simulink model "model1"  (R2024a)
settings: Solver=ode23t  StartTime=0.0  StopTime=finalatt{end,1}  MaxStep=0.1  RelTol=1e-3
undefined symbols (not defined in the file): finalatt, FrontAxle, FrontGear, MassWheel, NewData, RadiusWheel, RearAxle, RearGear, SlipAngle, TrackData, VehicleMass
libraries: fl_lib x16, batt_lib x13, nesl_utility x11, sdl_lib x7, ee_lib x2, simulink x1
(part 1 of 2)
settings Model: Creator=baiqu  LastModifiedBy=baiqu
settings SolverCC: MaxConsecutiveMinStep=5  ZeroCrossAlgorithm=Adaptive

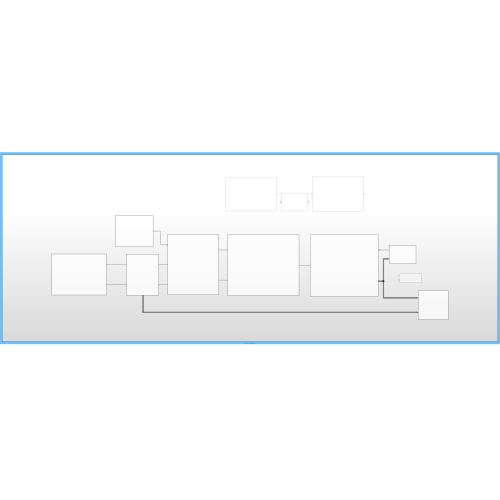
[thumbnail: Simulink's stored preview of the top-level diagram]
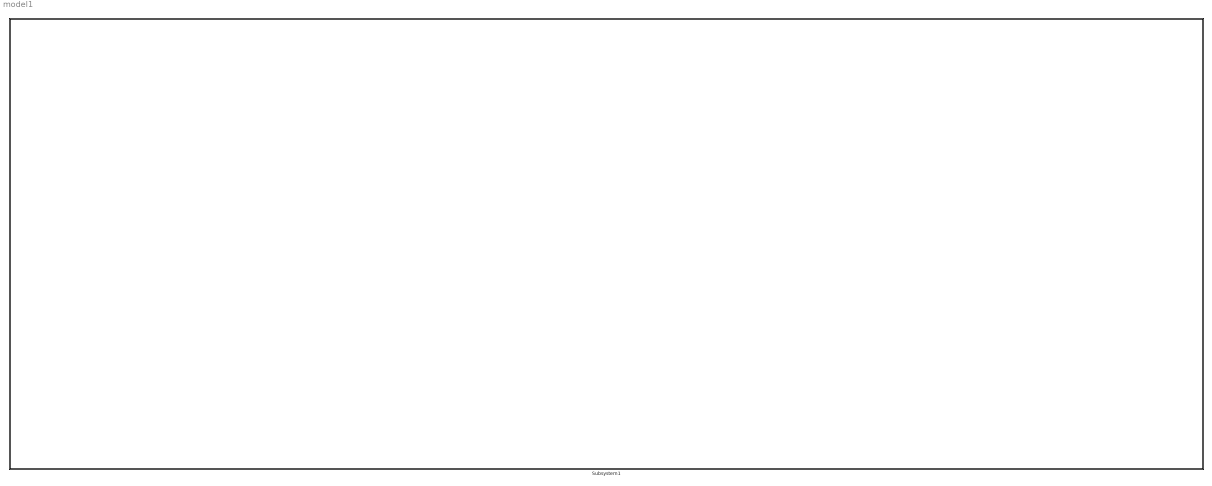
== system model1 ==
  Subsystem1 : Subsystem

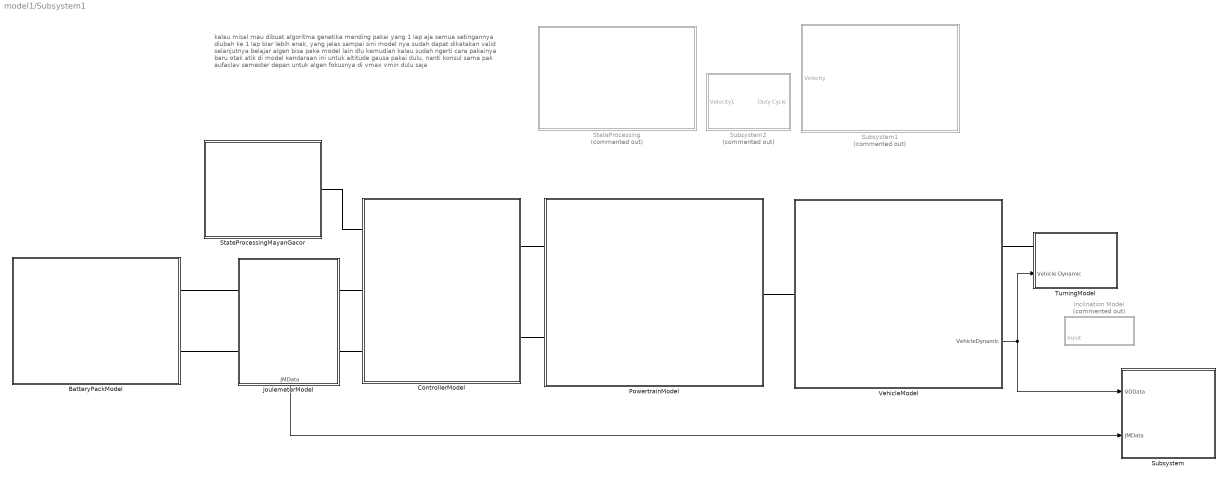
== system model1/Subsystem1 ==
  note: kalau misal mau dibuat algoritma genetika mending pakai yang 1 lap aja semua setingannya diubah ke 1 lap biar lebih enak, yang jelas sampai sini model nya sudah dapat dikatakan valid
      |
      | selanjutnya belajar algen bisa pake model lain dlu kemudian kalau sudah ngerti cara pakainya baru otak atik di model kendaraan ini
      |
      | untuk altitude gausa pakai dulu, nanti konsul sama pak aufaclav semester depan
      |
      | untuk algen fokusnya di vmax vmin dulu saja
  BatteryPackModel : Subsystem
  ControllerModel : Subsystem
  Inclination Model : Subsystem  Commented=on
      settings: PortSchema="{\"entries\":[{\"content\":{\"sides\":[{\"content\":{},\"type\":\"ConnectorPlacement.EquallySpacedRectSide\",\"uuid\":\"136e15b9-992d-4bd3-9ecd-22bc584851ec\"},{\"content\":{\"connectorIds\":[\"RConn1\",\"In1\"],\"side\":\"RIGHT\"},\"type\":\"ConnectorPlacement.EquallySpacedRectSide\",\"uuid\":\"21901198-73a1-4f2b-bd2a-55a4ec918fc9\"},{\"content\":{\"side\":\"TOP\"},\"type\":\"ConnectorPlacement.EquallySpacedRectSide\",\"uuid\":\"96b62914-b1ee-40c2-9187-7fe30b0e8d87\"}]},\"type\":\"ConnectorPlacement.EquallySpacedConnector\",\"uuid\":\"3de7d7f5-6cf3-49e2-811a-f65baadaba13\"}],\"packageUris\":[\"http://schema.mathworks.com/mf0/Connector/R2020b\"],\"version\":\"1.0\"}"
  JoulemeterModel : Subsystem
      settings: PortSchema="{\"entries\":[{\"content\":{\"sides\":[{\"content\":{\"connectorIds\":[\"LConn1\",\"LConn2\"]},\"type\":\"ConnectorPlacement.EquallySpacedRectSide\",\"uuid\":\"5b7f183a-bf7a-4999-b582-2617b2cbf3b5\"},{\"content\":{\"connectorIds\":[\"RConn1\",\"RConn2\"],\"side\":\"RIGHT\"},\"type\":\"ConnectorPlacement.EquallySpacedRectSide\",\"uuid\":\"60e6a297-a548-4f80-bd0a-fa1cc363ffaf\"},{\"content\":{\"side\":\"TOP\"},\"type\":\"ConnectorPlacement.EquallySpacedRectSide\",\"uuid\":\"7f0257a8-d3f8-4392-a80f-b293aa05a497\"},{\"content\":{\"connectorIds\":[\"Out1\"],\"side\":\"BOTTOM\"},\"type\":\"ConnectorPlacement.EquallySpacedRectSide\",\"uuid\":\"bc8eaeec-fb49-4b5e-9f30-46577002e429\"}]},\"type\":\"ConnectorPlacement.EquallySpacedConnector\",\"uuid\":\"4d471f89-f217-48cc-a8db-ea855d9b8dd6\"}],\"packageUris\":[\"http://schema.mathworks.com/mf0/Connector/R2020b\"],\"version\":\"1.0\"}"
  PowertrainModel : Subsystem
  StateProcessing : Subsystem  Commented=on
  StateProcessingMayanGacor : Subsystem
  Subsystem : Subsystem
  Subsystem1 : Subsystem  Commented=on
  Subsystem2 : Subsystem  Commented=on
  TurningModel : Subsystem
      settings: PortSchema="{\"entries\":[{\"content\":{\"sides\":[{\"content\":{\"connectorIds\":[\"LConn1\",\"In1\"]},\"type\":\"ConnectorPlacement.EquallySpacedRectSide\",\"uuid\":\"71e7bed3-e1e3-4832-b1c1-24de9e1463fb\"},{\"content\":{\"side\":\"RIGHT\"},\"type\":\"ConnectorPlacement.EquallySpacedRectSide\",\"uuid\":\"85b25ef4-cea1-4d54-8b2c-2c7e7889f274\"},{\"content\":{\"side\":\"TOP\"},\"type\":\"ConnectorPlacement.EquallySpacedRectSide\",\"uuid\":\"88c22c9a-8431-4448-acf4-309695bed040\"}]},\"type\":\"ConnectorPlacement.EquallySpacedConnector\",\"uuid\":\"9b68c14c-70b8-4970-8604-5181bbf23f66\"}],\"packageUris\":[\"http://schema.mathworks.com/mf0/Connector/R2020b\"],\"version\":\"1.0\"}"
  VehicleModel : Subsystem
      settings: PortSchema="{\"entries\":[{\"content\":{\"sides\":[{\"content\":{\"connectorIds\":[\"LConn1\"]},\"type\":\"ConnectorPlacement.EquallySpacedRectSide\",\"uuid\":\"dbac9918-d97a-4fb9-bcac-715c55eb3548\"},{\"content\":{\"connectorIds\":[\"RConn1\",\"Out1\"],\"side\":\"RIGHT\"},\"type\":\"ConnectorPlacement.EquallySpacedRectSide\",\"uuid\":\"c709c379-adcf-4afd-bad7-556514c49845\"},{\"content\":{\"side\":\"TOP\"},\"type\":\"ConnectorPlacement.EquallySpacedRectSide\",\"uuid\":\"0d093c29-8fc7-4ed3-9b38-7f716bf50260\"}]},\"type\":\"ConnectorPlacement.EquallySpacedConnector\",\"uuid\":\"a77c3579-3db4-497e-9cef-798accda3f16\"}],\"packageUris\":[\"http://schema.mathworks.com/mf0/Connector/R2020b\"],\"version\":\"1.0\"}"
  wires:
  JoulemeterModel/1(JMData) -> Subsystem/2(JMData)
  VehicleModel/1(VehicleDynamic) -> TurningModel/1(Vehicle Dynamic), Subsystem/1(VDData)
  connections:
  PowertrainModel/RConn1 -- VehicleModel/LConn1
  JoulemeterModel/LConn1 -- BatteryPackModel/RConn1
  ControllerModel/RConn1 -- PowertrainModel/LConn1
  JoulemeterModel/RConn2 -- ControllerModel/LConn3
  JoulemeterModel/RConn1 -- ControllerModel/LConn2
  PowertrainModel/LConn2 -- ControllerModel/RConn2
  BatteryPackModel/RConn2 -- JoulemeterModel/LConn2
  TurningModel/LConn1 -- VehicleModel/RConn1
  StateProcessingMayanGacor/RConn1 -- ControllerModel/LConn1

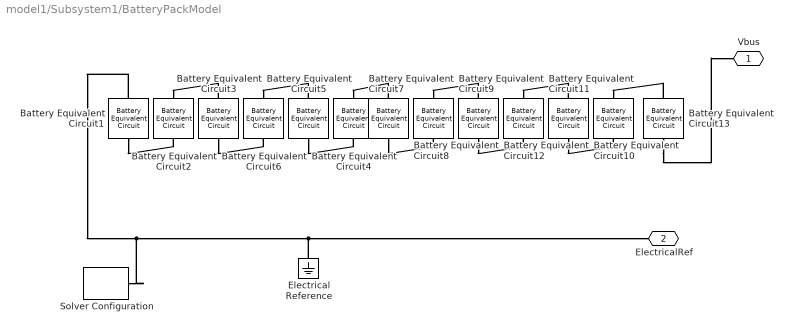
== system model1/Subsystem1/BatteryPackModel ==
  Battery Equivalent Circuit{1..13} (13 alike) : batt_lib/Cells/Battery Equivalent Circuit  Tag={'toolbox/physmod/battery/library/m/batt_lib_parts';'Cells/Battery_Equivalent_Circuit/Molicel/INR_21700_P45B.xml'}  BatteryCapacity=4.493 hr*A  ThermalModel=simscape.battery.enum.cells.BatteryThermalModel.ConstantTemperature  ExtrapolationMethod=simscape.enum.extrapolation.linear  EnableFaultExotherm=false % Parameter not set  TriggerTemperature=350 % Parameter not set K  SOCBreakpoints=[0 0.01 0.02 0.03 0.04 0.05 0.06 0.07 0.08 0.09 0.1 0.11 0.12 0.13 0.14 0.15 0.16 0.17 0.18 0.19 0.2 0.21 0.22 0.23 0.24 0.25 0.26 0.27 0.28 0.29 0.3 0.31 0.32 0.33 0.34 0.35 0.36 0.37 0.38 0.39 0.4 0.41 0.42 0.43 0.44 0.45 0.46 0.47 0.48 0.49 0.5 0.51 0.52 0.53 0.54 0.55 0.56 0.57 0.58 0.59 0.6 0.61 0.62 0.63 0.64 0.65 0.66 0.67 0.68 0.69 0.7 0.71 0.72 0.73 0.74 0.75 0.76 0.77 0.78 0.79 0.8 0.81 0.82 0.83 0.84 0.85 0.86 0.87 0.88 0.89 0.9 0.91 0.92 0.93 0.94 0.95 0.96 0.97 0.98 0.99 1]  TemperatureBreakpoints=[-40 -30 -20 0 23 45 60] degC  OpenCircuitVoltage=[3.17242 3.18272 3.19302 3.20331 3.21361 3.22391 3.23421 3.24451 3.25481 3.2651 3.2754 3.2857 3.296 3.3063 3.31659 3.32689 3.33719 3.34749 3.35779 3.36809 3.37838 3.38868 3.39898 3.40928 3.41958 3.42988 3.44017 3.45047 3.46077 3.47107 3.48137 3.49166 3.50196 3.51226 3.52256 3.53286 3.54316 3.55345 3.56375 3.57405 3.58435 3.59465 3.60495 3.61524 3.62554 3.63584 3.64614 3.65644 3.66673 3.67703 3.68733 3.69763 3.71041 3.72113 3.72997 3.73882 3.74912 3.75936 3.76951 3.7791 3.78865 3.79787 3.80709 3.8161 3.82509 3.83409 3.84308 3.85207 3.86107 3.87006 3.87901 3.88831 3.89824 3.90887 3.91951 3.93012 3.94073 3.95138 3.96184 3.97226 3.98268 3.99311 4.0032 4.01221 4.01944 4.02668 4.03286 4.03874 4.04383 4.0488 4.05377 4.05873 4.06312 4.06753 4.07333 4.08117 4.08904 4.09911 4.11111 4.13802 4.16831] V  OpenCircuitVoltageThermal=[3.17242 3.17242 3.17242 3.17242 3.17242 3.17242 3.17242;3.18272 3.18272 3.18272 3.18272 3.18272 3.18272 3.18272;3.19302 3.19302 3.19302 3.19302 3.19302 3.19302 3.19302;3.20331 3.20331 3.20331 3.20331 3.20331 3.20331 3.20331;3.21361 3.21361 3.21361 3.21361 3.21361 3.21361 3.21361;3.22391 3.22391 3.22391 3.22391 3.22391 3.22391 3.22391;3.23421 3.23421 3.23421 3.23421 3.23421 3.23421 3.23421;3.24451 3.24451 3.24451 3.24451 3.24451 3.24451 3.24451;3.25481 3.25481 3.25481 3.25481 3.25481 3.25481 3.25481;3.2651 3.2651 3.2651 3.2651 3.2651 3.2651 3.2651;3.2754 3.2754 3.2754 3.2754 3.2754 3.2754 3.2754;3.2857 3.2857 3.2857 3.2857 3.2857 3.2857 3.2857;3.296 3.296 3.296 3.296 3.296 3.296 3.296;3.3063 3.3063 3.3063 3.3063 3.3063 3.3063 3.3063;3.31659 3.31659 3.31659 3.31659 3.31659 3.31659 3.31659;3.32689 3.32689 3.32689 3.32689 3.32689 3.32689 3.32689;3.33719 3.33719 3.33719 3.33719 3.33719 3.33719 3.33719;3.34749 3.34749 3.34749 3.34749 3.34749 3.34749 3.34749;3.35779 3.35779 3.35779 3.35779 3.35779 3.35779 3.35779;3.36809 3.36809 3.36809 3.36809 3.36809 3.36809 3.36809;3.37838 3.37838 3.37838 3.37838 3.37838 3.37838 3.37838;3.38868 3.38868 3.38868 3.38868 3.38868 3.38868 3.38868;3.39898 3.39898 3.39898 3.39898 3.39898 3.39898 3.39898;3.40928 3.40928 3.40928 3.40928 3.40928 3.40928 3.40928;3.41958 3.41958 3.41958 3.41958 3.41958 3.41958 3.41958;3.42988 3.42988 3.42988 3.42988 3.42988 3.42988 3.42988;3.44017 3.44017 3.44017 3.44017 3.44017 3.44017 3.44017;3.45047 3.45047 3.45047 3.45047 3.45047 3.45047 3.45047;3.46077 3.46077 3.46077 3.46077 3.46077 3.46077 3.46077;3.47107 3.47107 3.47107 3.47107 3.47107 3.47107 3.47107;3.48137 3.48137 3.48137 3.48137 3.48137 3.48137 3.48137;3.49166 3.49166 3.49166 3.49166 3.49166 3.49166 3.49166;3.50196 3.50196 3.50196 3.50196 3.50196 3.50196 3.50196;3.51226 3.51226 3.51226 3.51226 3.51226 3.51226 3.51226;3.52256 3.52256 3.52256 3.52256 3.52256 3.52256 3.52256;3.53286 3.53286 3.53286 3.53286 3.53286 3.53286 3.53286;3.54316 3.54316 3.54316 3.54316 3.54316 3.54316 3.54316;3.55345 3.55345 3.55345 3.55345 3.55345 3.55345 3.55345;3.56375 3.56375 3.56375 3.56375 3.56375 3.56375 3.56375;3.57405 3.57405 3.57405 3.57405 3.57405 3.57405 3.57405;3.58435 3.58435 3.58435 3.58435 3.58435 3.58435 3.58435;3.59465 3.59465 3.59465 3.59465 3.59465 3.59465 3.59465;3.60495 3.60495 3.60495 3.60495 3.60495 3.60495 3.60495;3.61524 3.61524 3.61524 3.61524 3.61524 3.61524 3.61524;3.62554 3.62554 3.62554 3.62554 3.62554 3.62554 3.62554;3.63584 3.63584 3.63584 3.63584 3.63584 3.63584 3.63584;3.64614 3.64614 3.64614 3.64614 3.64614 3.64614 3.64614;3.65644 3.65644 3.65644 3.65644 3.65644 3.65644 3.65644;3.66673 3.66673 3.66673 3.66673 3.66673 3.66673 3.66673;3.67703 3.67703 3.67703 3.67703 3.67703 3.67703 3.67703;3.68733 3.68733 3.68733 3.68733 3.68733 3.68733 3.68733;3.69763 3.69763 3.69763 3.69763 3.69763 3.69763 3.69763;3.71041 3.71041 3.71041 3.71041 3.71041 3.71041 3.71041;3.72113 3.72113 3.72113 3.72113 3.72113 3.72113 3.72113;3.72997 3.72997 3.72997 3.72997 3.72997 3.72997 3.72997;3.73882 3.73882 3.73882 3.73882 3.73882 3.73882 3.73882;3.74912 3.74912 3.74912 3.74912 3.74912 3.74912 3.74912;3.75936 3.75936 3.75936 3.75936 3.75936 3.75936 3.75936;3.76951 3.76951 3.76951 3.76951 3.76951 3.76951 3.76951;3.7791 3.7791 3.7791 3.7791 3.7791 3.7791 3.7791;3.78865 3.78865 3.78865 3.78865 3.78865 3.78865 3.78865;3.79787 3.79787 3.79787 3.79787 3.79787 3.79787 3.79787;3.80709 3.80709 3.80709 3.80709 3.80709 3.80709 3.80709;3.8161 3.8161 3.8161 3.8161 3.8161 3.8161 3.8161;3.82509 3.82509 3.82509 3.82509 3.82509 3.82509 3.82509;3.83409 3.83409 3.83409 3.83409 3.83409 3.83409 3.83409;3.84308 3.84308 3.84308 3.84308 3.84308 3.84308 3.84308;3.85207 3.85207 3.85207 3.85207 3.85207 3.85207 3.85207;3.86107 3.86107 3.86107 3.86107 3.86107 3.86107 3.86107;3.87006 3.87006 3.87006 3.87006 3.87006 3.87006 3.87006;3.87901 3.87901 3.87901 3.87901 3.87901 3.87901 3.87901;3.88831 3.88831 3.88831 3.88831 3.88831 3.88831 3.88831;3.89824 3.89824 ...(+1594 chars)] V  VoltageRange=[2.25 Inf] V  HysteresisModel=simscape.battery.enum.cells.HysteresisModel.none  MaximumHysteresisVoltage=[0, 0, 0, 0, 0, 0, 0] % Parameter not set V  InstantaneousHysteresisVoltage=[0, 0, 0, 0, 0, 0, 0] % Parameter not set V  HysteresisRate=0.1 % Parameter not set  MaximumHysteresisVoltageThermal=[0, 0, 0; 0, 0, 0; 0, 0, 0; 0, 0, 0; 0, 0, 0; 0, 0, 0; 0, 0, 0] % Parameter not set V  InstantaneousHysteresisVoltageThermal=[0, 0, 0; 0, 0, 0; 0, 0, 0; 0, 0, 0; 0, 0, 0; 0, 0, 0; 0, 0, 0] % Parameter not set V  HysteresisRateThermal=0.1 % Parameter not set  ResistanceSOCBreakpoints=[0 0.01 0.02 0.03 0.04 0.05 0.06 0.07 0.08 0.09 0.1 0.11 0.12 0.13 0.14 0.15 0.16 0.17 0.18 0.19 0.2 0.21 0.22 0.23 0.24 0.25 0.26 0.27 0.28 0.29 0.3 0.31 0.32 0.33 0.34 0.35 0.36 0.37 0.38 0.39 0.4 0.41 0.42 0.43 0.44 0.45 0.46 0.47 0.48 0.49 0.5 0.51 0.52 0.53 0.54 0.55 0.56 0.57 0.58 0.59 0.6 0.61 0.62 0.63 0.64 0.65 0.66 0.67 0.68 0.69 0.7 0.71 0.72 0.73 0.74 0.75 0.76 0.77 0.78 0.79 0.8 0.81 0.82 0.83 0.84 0.85 0.86 0.87 0.88 0.89 0.9 0.91 0.92 0.93 0.94 0.95 0.96 0.97 0.98 0.99 1]  ResistanceTemperatureBreakpoints=[-40 -30 -20 0 23 45 60] degC  CurrentDirectionality=simscape.battery.enum.cells.BatteryEnable.Disabled  R0=[0.02095 0.01921 0.01774 0.0166 0.01557 0.01469 0.01398 0.01338 0.01283 0.01239 0.01196 0.01155 0.01116 0.01079 0.01042 0.01007 0.00974 0.00949 0.00924 0.009 0.00876 0.00855 0.00843 0.00832 0.00826 0.00825 0.00825 0.00826 0.00827 0.00828 0.0083 0.00834 0.00838 0.00842 0.00848 0.00855 0.00863 0.00871 0.00879 0.00887 0.00895 0.00903 0.00911 0.00918 0.00925 0.00931 0.00938 0.00946 0.00953 0.00961 0.00968 0.00976 0.00991 0.01 0.01003 0.01006 0.01013 0.01022 0.0103 0.01037 0.01043 0.01049 0.01055 0.01061 0.01066 0.01072 0.01077 0.01082 0.01088 0.01093 0.01099 0.01105 0.01114 0.01125 0.01136 0.01148 0.01161 0.01175 0.01188 0.01202 0.01215 0.01228 0.01241 0.01253 0.01261 0.01269 0.01275 0.0128 0.01285 0.01289 0.01294 0.01298 0.01296 0.01292 0.01292 0.01288 0.01282 0.0128 0.01232 0.01214 0.00952] Ohm  R0Thermal=[0.3026 0.35142 0.34349 0.24415 0.02095 0.15874 0.14729;0.2941 0.33555 0.32379 0.22614 0.01921 0.13363 0.12249;0.28559 0.31969 0.30408 0.20813 0.01774 0.10853 0.10276;0.27709 0.30382 0.28438 0.19012 0.0166 0.09423 0.0861;0.26858 0.28796 0.26468 0.17211 0.01557 0.07998 0.0748;0.26008 0.27209 0.24498 0.1541 0.01469 0.07024 0.06679;0.25157 0.25623 0.22527 0.1361 0.01398 0.06387 0.05877;0.24307 0.24036 0.20557 0.11861 0.01338 0.0575 0.05275;0.23456 0.2245 0.18587 0.10674 0.01283 0.05113 0.04899;0.22606 0.20863 0.16617 0.09525 0.01239 0.04679 0.04522;0.21755 0.19277 0.14651 0.08799 0.01196 0.0439 0.04145;0.20905 0.1769 0.13098 0.08073 0.01155 0.04101 0.03817;0.20054 0.16103 0.11905 0.07347 0.01116 0.03813 0.03522;0.19204 0.14769 0.11102 0.06895 0.01079 0.03524 0.03228;0.18353 0.13913 0.10517 0.06499 0.01042 0.03235 0.02934;0.17503 0.13157 0.09933 0.06104 0.01007 0.02946 0.0264;0.16653 0.1271 0.09371 0.05708 0.00974 0.02657 0.02345;0.15804 0.12264 0.09094 0.05312 0.00949 0.02417 0.02125;0.15354 0.11817 0.08816 0.04917 0.00924 0.02286 0.01972;0.14976 0.11385 0.08539 0.04748 0.009 0.02156 0.0182;0.14598 0.11213 0.08261 0.04617 0.00876 0.02025 0.01667;0.14219 0.11042 0.08103 0.04487 0.00855 0.01894 0.01515;0.14033 0.10871 0.08035 0.04356 0.00843 0.01763 0.01363;0.13876 0.10699 0.07967 0.04225 0.00832 0.01632 0.0121;0.13718 0.10528 0.07899 0.04094 0.00826 0.01501 0.01058;0.13561 0.10357 0.07831 0.03964 0.00825 0.0137 0.00906;0.13404 0.10198 0.07763 0.03833 0.00825 0.01239 0.00753;0.13247 0.10119 0.07695 0.03702 0.00826 0.01108 0.0065;0.13096 0.10039 0.07627 0.03624 0.00827 0.00977 0.00633;0.13043 0.0996 0.07559 0.03615 0.00828 0.00846 0.00617;0.1299 0.0988 0.07491 0.03606 0.0083 0.00774 0.006;0.12937 0.09801 0.07423 0.03597 0.00834 0.00779 0.00583;0.12883 0.09721 0.07355 0.03588 0.00838 0.00783 0.00567;0.1283 0.09642 0.07301 0.03579 0.00842 0.00787 0.0055;0.12777 0.09585 0.07296 0.0357 0.00848 0.00792 0.00534;0.12724 0.09584 0.07291 0.03561 0.00855 0.00796 0.00517;0.12675 0.09584 0.07286 0.03552 0.00863 0.00801 0.005;0.12643 0.09583 0.0728 0.03543 0.00871 0.00805 0.00484;0.12611 0.09582 0.07275 0.03534 0.00879 0.00809 0.00467;0.12579 0.09582 0.0727 0.03525 0.00887 0.00814 0.0045;0.12547 0.09581 0.07264 0.03526 0.00895 0.00818 0.00434;0.12514 0.0958 0.07259 0.03537 0.00903 0.00823 0.00405;0.12482 0.09579 0.07254 0.03547 0.00911 0.00804 0.00366;0.1245 0.09579 0.07248 0.03558 0.00918 0.00776 0.00327;0.12418 0.09578 0.07243 0.03568 0.00925 0.00748 0.00287;0.12386 0.09577 0.07231 0.03579 0.00931 0.0072 0.00248;0.12354 0.09576 0.0721 0.03589 0.00938 0.00692 0.00209;0.12322 0.09576 0.07189 0.036 0.00946 0.00664 0.0017;0.12301 0.09575 0.07168 0.03611 0.00953 0.00636 0.00131;0.12309 0.09574 0.07147 0.03621 0.00961 0.00608 0.00092;0.12318 0.09573 0.07125 0.0363 0.00968 0.0058 0.00053;0.12326 0.09573 0.07104 0.03637 0.00976 0.00552 0.00014;0.12389 0.09628 0.07138 0.03699 0.00991 0.00579 0.0003;0.12407 0.09637 0.07126 0.03715 0.01 0.0056 0.0003;0.12383 0.09605 0.07073 0.0369 0.01003 0.00504 0.0003;0.12359 0.09573 0.07019 0.03664 0.01006 0.00503 0.0003;0.12367 0.09573 0.06998 0.03671 0.01013 0.00534 0.00063;0.12375 0.09572 0.06975 0.03677 0.01022 0.00564 0.00094;0.1238 0.09569 0.07006 0.0368 0.0103 0.00593 0.00123;0.12372 0.09554 0.07026 0.03671 0.01037 0.00608 0.00139;0.12364 0.09537 0.07046 0.03661 0.01043 0.00623 0.00155;0.12348 0.09514 0.07058 0.03644 0.01049 0.0063 0.00163;0.12333 0.0949 0.07071 0.03627 0.01055 0.00638 0.00171;0.12312 0.09461 0.07078 0.03605 0.01061 0.00641 0.00175;0.12291 0.09433 0.07085 0.03583 0.01066 0.00643 0.00168;0.12271 0.09404 0.07093 0.03568 0.01072 0.00646 0.00161;0.12275 0.09398 0.071 0.03622 0.01077 0.00646 0.00153;0.12316 0.09449 0.07107 0.03677 0.01082 0.00636 0.00145;0.12357 0.095 0.07115 0.03731 0.01088 0.00625 0.00137;0.12398 0.09551 0.07151 0.03785 0.01093 0.00614 0.00129;0.12438 0.09601 0.07221 0.03839 0.01099 0.00602 0.0012;0.12486 0.09659 0.07299 0.039 0.01105 0.00599 0.00119;0.12548 0.09731 0.07391 ...(+1579 chars)] Ohm  DischargeR0=[.0085, .0085, .0087, .0082, .0083, .0085, .0085] % Parameter not set Ohm  ChargeR0=[.0085, .0085, .0087, .0082, .0083, .0085, .0085] % Parameter not set Ohm  ChargeR0Thermal=[.0117, .0085, .009; .011, .0085, .009; .0114, .0087, .0092; .0107, .0082, .0088; .0107, .0083, .0091; .0113, .0085, .0089; .0116, .0085, .0089] % Parameter not set Ohm  DischargeR0Thermal=[.0117, .0085, .009; .011, .0085, .009; .0114, .0087, .0092; .0107, .0082, .0088; .0107, .0083, .0091; .0113, .0085, .0089; .0116, .0085, .0089] % Parameter not set Ohm  SelfDischargeResistor=simscape.battery.enum.cells.BatteryEnable.Disabled  SelfDischargeR=7e3 % Parameter not set Ohm  SelfDischargeRThermal=[8000, 7000, 6000] % Parameter not set Ohm  RCPairs=simscape.battery.enum.cells.RCPairs.noDynamics  R1=[.0029, .0024, .0026, .0016, .0023, .0018, .0017] % Parameter not set Ohm  Tau1=[36, 45, 105, 29, 77, 33, 39] % Parameter not set s  R2=[.0029, .0024, .0026, .0016, .0023, .0018, .0017] % Parameter not set Ohm  Tau2=[36, 45, 105, 29, 77, 33, 39] % Parameter not set s  R3=[.0029, .0024, .0026, .0016, .0023, .0018, .0017] % Parameter not set Ohm  Tau3=[36, 45, 105, 29, 77, 33, 39] % Parameter not set s  DischargeR1=[.0029, .0024, .0026, .0016, .0023, .0018, .0017] % Parameter not set Ohm  DischargeTau1=[36, 45, 105, 29, 77, 33, 39] % Parameter not set s  ChargeR1=[.0029, .0024, .0026, .0016, .0023, .0018, .0017] % Parameter not set Ohm  ChargeTau1=[36, 45, 105, 29, 77, 33, 39] % Parameter not set s  DischargeR2=[.0029, .0024, .0026, .0016, .0023, .0018, .0017] % Parameter not set Ohm  DischargeTau2=[36, 45, 105, 29, 77, 33, 39] % Parameter not set s  ChargeR2=[.0029, .0024, .0026, .0016, .0023, .0018, .0017] % Parameter not set Ohm  ChargeTau2=[36, 45, 105, 29, 77, 33, 39] % Parameter not set s  DischargeR3=[.0029, .0024, .0026, .0016, .0023, .0018, .0017] % Parameter not set Ohm  DischargeTau3=[36, 45, 105, 29, 77, 33, 39] % Parameter not set s  ChargeR3=[.0029, .0024, .0026, .0016, .0023, .0018, .0017] % Parameter not set Ohm  ChargeTau3=[36, 45, 105, 29, 77, 33, 39] % Parameter not set s  R1Thermal=[.0109, .0029, .0013; .0069, .0024, .0012; .0047, .0026, .0013; .0034, .0016, .001; .0033, .0023, .0014; .0033, .0018, .0011; .0028, .0017, .0011] % Parameter not set Ohm  Tau1Thermal=[20, 36, 39; 31, 45, 39; 109, 105, 61; 36, 29, 26; 59, 77, 67; 40, 33, 29; 25, 39, 33] % Parameter not set s  R2Thermal=[.0109, .0029, .0013; .0069, .0024, .0012; .0047, .0026, .0013; .0034, .0016, .001; .0033, .0023, .0014; .0033, .0018, .0011; .0028, .0017, .0011] % Parameter not set Ohm  Tau2Thermal=[20, 36, 39; 31, 45, 39; 109, 105, 61; 36, 29, 26; 59, 77, 67; 40, 33, 29; 25, 39, 33] % Parameter not set s  R3Thermal=[.0109, .0029, .0013; .0069, .0024, .0012; .0047, .0026, .0013; .0034, .0016, .001; .0033, .0023, .0014; .0033, .0018, .0011; .0028, .0017, .0011] % Parameter not set Ohm  Tau3Thermal=[20, 36, 39; 31, 45, 39; 109, 105, 61; 36, 29, 26; 59, 77, 67; 40, 33, 29; 25, 39, 33] % Parameter not set s  DischargeR1Thermal=[.0109, .0029, .0013; .0069, .0024, .0012; .0047, .0026, .0013; .0034, .0016, .001; .0033, .0023, .0014; .0033, .0018, .0011; .0028, .0017, .0011] % Parameter not set Ohm  DischargeTau1Thermal=[20, 36, 39; 31, 45, 39; 109, 105, 61; 36, 29, 26; 59, 77, 67; 40, 33, 29; 25, 39, 33] % Parameter not set s  ChargeR1Thermal=[.0109, .0029, .0013; .0069, .0024, .0012; .0047, .0026, .0013; .0034, .0016, .001; .0033, .0023, .0014; .0033, .0018, .0011; .0028, .0017, .0011] % Parameter not set Ohm  ChargeTau1Thermal=[20, 36, 39; 31, 45, 39; 109, 105, 61; 36, 29, 26; 59, 77, 67; 40, 33, 29; 25, 39, 33] % Parameter not set s  DischargeR2Thermal=[.0109, .0029, .0013; .0069, .0024, .0012; .0047, .0026, .0013; .0034, .0016, .001; .0033, .0023, .0014; .0033, .0018, .0011; .0028, .0017, .0011] % Parameter not set Ohm  DischargeTau2Thermal=[20, 36, 39; 31, 45, 39; 109, 105, 61; 36, 29, 26; 59, 77, 67; 40, 33, 29; 25, 39, 33] % Parameter not set s  ChargeR2Thermal=[.0109, .0029, .0013; .0069, .0024, .0012; .0047, .0026, .0013; .0034, .0016, .001; .0033, .0023, .0014; .0033, .0018, .0011; .0028, .0017, .0011] % Parameter not set Ohm  ChargeTau2Thermal=[20, 36, 39; 31, 45, 39; 109, 105, 61; 36, 29, 26; 59, 77, 67; 40, 33, 29; 25, 39, 33] % Parameter not set s  DischargeR3Thermal=[.0109, .0029, .0013; .0069, .0024, .0012; .0047, .0026, .0013; .0034, .0016, .001; .0033, .0023, .0014; .0033, .0018, .0011; .0028, .0017, .0011] % Parameter not set Ohm  DischargeTau3Thermal=[20, 36, 39; 31, 45, 39; 109, 105, 61; 36, 29, 26; 59, 77, 67; 40, 33, 29; 25, 39, 33] % Parameter not set s  ChargeR3Thermal=[.0109, .0029, .0013; .0069, .0024, .0012; .0047, .0026, .0013; .0034, .0016, .001; .0033, .0023, .0014; .0033, .0018, .0011; .0028, .0017, .0011] % Parameter not set Ohm  ChargeTau3Thermal=[20, 36, 39; 31, 45, 39; 109, 105, 61; 36, 29, 26; 59, 77, 67; 40, 33, 29; 25, 39, 33] % Parameter not set s  CyclingAgingMethod=simscape.battery.enum.cells.CyclingAgingMethod.tableN  NumDisCycles=100 % Parameter not set  OCVChange=0 % Parameter not set  R0Change=0 % Parameter not set  CapacityChange=0 % Parameter not set  SelfDischargeRChange=0 % Parameter not set  R1Change=0 % Parameter not set  R2Change=0 % Parameter not set  R3Change=0 % Parameter not set  NumDisCyclesBreakpoints=[0 6 11 16 21 26 31 36 41 46 51 56 61 66 71 76 81 86 91 96 101 106 111 116 121 126 131 136 141 146 151 156 161 166 171 176 181 186 191 196 201 206 211 216 221 226 231 236 241 246 251 256 261 266 271 276 281 286 291 296 301 306 311 316 321 326 331 336 341 346 351 356 361 366 371 376 381 386 391 396 401 406 411 416 421 426 431 436 441 446 451 456 461 466 471 476 481 486 491 496]  AgingTemperatureBreakpoints=[298.15, 323.15] % Parameter not set K  OCVChangeVec=[0 -0.0674 -0.1349 -0.2023 -0.2697 -0.3371 -0.4046 -0.472 -0.5394 -0.6069 -0.6828 -0.7561 -0.8245 -0.8929 -0.9613 -1.0297 -1.0981 -1.1664 -1.2348 -1.3032 -1.3773 -1.4186 -1.4598 -1.5011 -1.5424 -1.5836 -1.6249 -1.6652 -1.6999 -1.7345 -1.7691 -1.8038 -1.8384 -1.8731 -1.908 -1.9398 -1.9715 -2.0033 -2.0351 -2.0669 -2.0986 -2.1303 -2.162 -2.1976 -2.2332 -2.2687 -2.2977 -2.3239 -2.3502 -2.3765 -2.4028 -2.4264 -2.4464 -2.4663 -2.4863 -2.5063 -2.5263 -2.5462 -2.5661 -2.5849 -2.6031 -2.6212 -2.6407 -2.6612 -2.6817 -2.7022 -2.7227 -2.7432 -2.7637 -2.7842 -2.8047 -2.8253 -2.8458 -2.8662 -2.8858 -2.9054 -2.9249 -2.9445 -2.9641 -2.9837 -3.0037 -3.0238 -3.0439 -3.064 -3.0841 -3.1042 -3.1267 -3.1499 -3.1731 -3.1989 -3.2248 -3.2508 -3.2781 -3.3053 -3.3326 -3.3598 -3.387 -3.4171 -3.449 -3.4809]  R0ChangeVec=[0 0 0 0 0 0 0 0 0 0 0 0 0 0 0 0 0 0 0 0 0 0 0 0 0 0 0 0 0 0 0 0 0 0 0 0 0 0 0 0 0 0 0 0 0 0 0 0 0 0 0 0 0 0 0 0 0 0 0 0 0 0 0 0 0 0 0 0 0 0 0 0 0 0 0 0 0 0 0 0 0 0 0 0 0 0 0 0 0 0 0 0 0 0 0 0 0 0 0 0] % Parameter assumed  CapacityChangeVec=[0 -0.093 -0.186 -0.278 -0.371 -0.464 -0.557 -0.649 -0.742 -0.835 -0.94 -1.045 -1.151 -1.257 -1.363 -1.469 -1.575 -1.681 -1.787 -1.893 -2.017 -2.161 -2.304 -2.447 -2.591 -2.734 -2.877 -3.021 -3.164 -3.307 -3.451 -3.594 -3.737 -3.881 -4.032 -4.201 -4.369 -4.538 -4.706 -4.874 -5.043 -5.211 -5.38 -5.569 -5.758 -5.947 -6.135 -6.324 -6.513 -6.702 -6.891 -7.08 -7.269 -7.458 -7.647 -7.836 -8.025 -8.214 -8.403 -8.582 -8.754 -8.927 -9.099 -9.271 -9.443 -9.615 -9.787 -9.96 -10.132 -10.304 -10.476 -10.648 -10.82 -10.992 -11.156 -11.32 -11.485 -11.649 -11.814 -11.978 -12.143 -12.307 -12.471 -12.636 -12.8 -12.965 -13.129 -13.293 -13.458 -13.641 -13.825 -14.008 -14.192 -14.376 -14.56 -14.743 -14.927 -15.111 -15.295 -15.478]  SelfDischargeRChangeVec=[0, 0, 0, 0] % Parameter not set  R1ChangeVec=[0, 0, 0, 0] % Parameter not set  R2ChangeVec=[0, 0, 0, 0] % Parameter not set  R3ChangeVec=[0, 0, 0, 0] % Parameter not set  OCVChangeThermal=[0, 0; 0, 0; 0, 0; 0, 0] % Parameter not set  R0ChangeThermal=[0, 0; 0, 0; 0, 0; 0, 0] % Parameter not set  CapacityChangeThermal=[0, 0; 0, 0; 0, 0; 0, 0] % Parameter not set  SelfDischargeRChangeThermal=[0, 0; 0, 0; 0, 0; 0, 0] % Parameter not set  R1ChangeThermal=[0, 0; 0, 0; 0, 0; 0, 0] % Parameter not set  R2ChangeThermal=[0, 0; 0, 0; 0, 0; 0, 0] % Parameter not set  R3ChangeThermal=[0, 0; 0, 0; 0, 0; 0, 0] % Parameter not set  CalendarAgeResistance=simscape.battery.enum.cells.BatteryEnable.Disabled  CalendarAgeCapacity=simscape.battery.enum.cells.BatteryEnable.Disabled  CalendarAgingMethod=simscape.battery.enum.cells.CalendarAgingMethod.equation  StorageVariable=simscape.battery.enum.cells.StorageVariable.OCV  OCVDuringStorage=0.9 % Parameter not set  SOCDuringStorage=0.6 % Parameter not set  StorageTimeIntervals=[0] % Parameter not set d  StorageTemperatures=[273] % Parameter not set K  ResistanceScalingOCV=2.2134e6 % Parameter not set  ResistanceScalingOCVOffset=1.632e6 % Parameter not set  ResistanceExponentialIncrease=0.515833569 % Parameter not set V  ResistanceTimeExponent=0.75 % Parameter not set  ResistanceAgeTemperatureBreakpoints=[273.15, 298.15, 323.15] % Parameter not set K  ResistanceAgeTimeBreakpoints=[0, 90, 180, 270] % Parameter not set d  PercentResistanceChange=[0, 0, 0] % Parameter not set  ResistanceTimeBreakpoints=100 % Parameter not set d  PercentResistanceChangeThermal=[0, 0, 0; 0, 0, 0; 0, 0, 0; 0, 0, 0] % Parameter not set  CapacityScalingOCV=1.5097e07 % Parameter not set  CapacityScalingOCVOffset=8.3625e06 % Parameter not set  CapacityExponentialIncrease=0.6011 % Parameter not set V  CapacityTimeExponent=0.75 % Parameter not set  CapacityAgeTemperatureBreakpoints=[273.15, 298.15, 323.15] % Parameter not set K  CapacityAgeTimeBreakpoints=[0, 90, 180, 270] % Parameter not set d  PercentCapacityChange=[0, 0, 0] % Parameter not set  CapacityTimeBreakpoints=100 % Parameter not set d  PercentCapacityChangeThermal=[0, 0, 0; 0, 0, 0; 0, 0, 0; 0, 0, 0] % Parameter not set  SimulationTemperature=298.15 % Parameter not set K  BatteryThermalMass=63 % Parameter assumed J/K  ReversibleHeatModel=simscape.battery.enum.cells.ReversibleHeatModel.Disabled  EntropicCoefficient=[0, 0, 0, 0, 0, 0, 0] % Parameter not set mV/K  AddedResistance=1e5 % Parameter not set Ohm  ShortedResistance=1e-6 % Parameter not set Ohm  ExothermModel=simscape.battery.enum.cells.ExothermModel.analytical  TabulateWithSOC=false % Parameter not set  SOCvecExotherm=[0, .5, 1] % Parameter not set  CurrInterruptTempSOC=[420, 420, 420] % Parameter not set K  TotalHeatOfReactionSOC=[23000, 23000, 23000] % Parameter not set J  CurrentInterruptTemperature=420 % Parameter not set K  TotalHeatOfReaction=23e3 % Parameter not set J  ExothermOnsetTemperature=350 % Parameter not set K  ExothermOnsetTempSOC=[350, 350, 350] % Parameter not set K  OnsetTempRate=0.02 % Parameter not set K/min  ActivationEnergy=160e3 % Parameter not set J/mol  ActivationEnergySOC=[160000, 160000, 160000] % Parameter not set J/mol  ReactionOrder=1 % Parameter not set  ReactionOrderSOC=[1, 1, 1] % Parameter not set  TemperaturesFromARC=[323, 373, 423, 438, 463, 483, 513, 543, 545, 547, 549, 551, 553, 573, 623, 773, 923, 943, 1003, 1063, 1113, 1123, 1133, 1153, 1173] % Parameter not set K  TemperatureRatesFromARC=[.0001, .001, .025, .2, .4, .6, 1.1, 1.3, 1.9, 3, 5, 11.6, 183.3, 191.6, 200, 208.3, 200, 175, 8.33, 1.33, .33, .2, .13, .0017, .00017] % Parameter not set K/s  TempRateVecARCSOC=repmat([.0001, .001, .025, .2, .4, .6, 1.1, 1.3, 1.9, 3, 5, 11.6, 183.3, 191.6, 200, 208.3, 200, 175, 8.33, 1.33, .33, .2, .13, .0017, .00017]', 1, 3) % Parameter not set K/s  PercentThermalMassVented=40 % Parameter not set  PercentThermalMassVentedSOC=[40, 40, 40] % Parameter not set  EnableFaultAddRes=false % Parameter not set  EnableFaultShort=false % Parameter not set  faultTriggerType=simscape.fault.triggertype.external % Parameter not set  stateOfCharge_specify=off  stateOfCharge_priority=High  stateOfCharge=1  stateOfCharge_nominal_specify=off  stateOfCharge_nominal_value=1  stateOfCharge_nominal_unit=1  numCycles_specify=off  numCycles_priority=High  numCycles=0  numCycles_nominal_specify=off  numCycles_nominal_value=1  numCycles_nominal_unit=1  batteryVoltage_specify=off  batteryVoltage_priority=None  batteryVoltage=0 V  batteryVoltage_nominal_specify=off  batteryVoltage_nominal_value=1  batteryVoltage_nominal_unit=V  batteryCurrent_specify=off  batteryCurrent_priority=None  batteryCurrent=0 A  batteryCurrent_nominal_specify=off  batteryCurrent_nominal_value=1  batteryCurrent_nominal_unit=A  batteryTemperature_specify=off  batteryTemperature_priority=High  batteryTemperature=298.15 K  batteryTemperature_nominal_specify=off  batteryTemperature_nominal_value=1  batteryTemperature_nominal_unit=K  hysteresisState_specify=off  hysteresisState_priority=High  hysteresisState=0  hysteresisState_nominal_specify=off  hysteresisState_nominal_value=1  hysteresisState_nominal_unit=1  isExothermFaulted_specify=off  isExothermFaulted_priority=None  isExothermFaulted=0  isExothermFaulted_nominal_specify=off  isExothermFaulted_nominal_value=1  isExothermFaulted_nominal_unit=1  isCurrentInterruptionTempExceeded_specify=off  isCurrentInterruptionTempExceeded_priority=None  isCurrentInterruptionTempExceeded=0  isCurrentInterruptionTempExceeded_nominal_specify=off  isCurrentInterruptionTempExceeded_nominal_value=1  isCurrentInterruptionTempExceeded_nominal_unit=1  reactionHeatRate_specify=off  reactionHeatRate_priority=None  reactionHeatRate=0 W  reactionHeatRate_nominal_specify=off  reactionHeatRate_nominal_value=1  reactionHeatRate_nominal_unit=W  reactionExtent_specify=off  reactionExtent_priority=None  reactionExtent=0  reactionExtent_nominal_specify=off  reactionExtent_nominal_value=1  reactionExtent_nominal_unit=1
      settings: AttributesFormatString=Molicel:INR_21700_P45B  InternalSimscapePortConfiguration="{\"Bottom\":[],\"Left\":[{\"id\":\"p\",\"label\":\"+\",\"type\":\"foundation.electrical.electrical\"}],\"Right\":[{\"id\":\"n\",\"label\":\"-\",\"type\":\"foundation.electrical.electrical\"}],\"Top\":[]}"
  Electrical Reference : fl_lib/Electrical/Electrical Elements/Electrical Reference
  Solver Configuration : nesl_utility/Solver Configuration  PhysicalDomain=network_engine_domain  SubClassName=solver  LeftPortType=input  RightPortType=generic  Tones=[]  Harmonics=[]  SimulateNoise=off  Profile=off  UseLocalSampling=off  EnableSwitchedLinearOptims=on  FrequencyDomain=off  UseCCode=off  RelTol=0.001  AbsTol=1e-06  MinStep=1e-09  ToWorkspace=off  RevertToSquareIcSolve=off  NumHomotopyIterations=100  PhasorMode=off  PhasorModeNumHarmonics=1  ConsistencySolver=NEWTON_FTOL  IndexReductionMethod=DerivativeReplacement  DoDC=off  ResidualTolerance=1e-09  ConsistencyTolSource=GLOBAL  ConsistencyAbsTol=0.001  ConsistencyRelTol=0.001  ConsistencyTolFactor=0.001  UseLocalSolver=off  LocalSolverChoice=NE_BACKWARD_EULER_ADVANCER  ResolveIndetEquations=on  FunctionEvalNumThread=1  LocalSolverSampleTime=0.001  DoFixedCost=on  MaxNonlinIter=10  MaxModeIter=2  ComputeImpulses=off  ImpulseIterations=2  LinearAlgebra=auto  LinearAlgebraNumThread=0  EquationFormulation=NE_TIME_EF  DelaysMemoryBudget=1024  AutomaticFiltering=on  FilteringTimeConstant=0.001  PartitionStorageMethod=AS_NEEDED  PartitionMemoryBudget=1024  PartitionMethod=ROBUST  MultibodyUseLocalSolver=off  MultibodyLocalSolverChoice=ODE1  MultibodyLocalSolverSampleTime=0.001
  Vbus : PMIOPort  Side=Right
  ElectricalRef : PMIOPort  Port=2  Side=Right
  connections:
  Solver Configuration/RConn1 -- ElectricalRef/RConn1 -- Electrical Reference/LConn1 -- Battery Equivalent Circuit1/RConn1
  Battery Equivalent Circuit1/LConn1 -- Battery Equivalent Circuit2/RConn1
  Battery Equivalent Circuit3/LConn1 -- Battery Equivalent Circuit6/RConn1
  Battery Equivalent Circuit5/LConn1 -- Battery Equivalent Circuit4/RConn1
  Battery Equivalent Circuit7/LConn1 -- Battery Equivalent Circuit8/RConn1
  Battery Equivalent Circuit9/LConn1 -- Battery Equivalent Circuit12/RConn1
  Battery Equivalent Circuit11/LConn1 -- Battery Equivalent Circuit10/RConn1
  Battery Equivalent Circuit13/LConn1 -- Vbus/RConn1
  Battery Equivalent Circuit13/RConn1 -- Battery Equivalent Circuit10/LConn1
  Battery Equivalent Circuit11/RConn1 -- Battery Equivalent Circuit12/LConn1
  Battery Equivalent Circuit9/RConn1 -- Battery Equivalent Circuit8/LConn1
  Battery Equivalent Circuit7/RConn1 -- Battery Equivalent Circuit4/LConn1
  Battery Equivalent Circuit5/RConn1 -- Battery Equivalent Circuit6/LConn1
  Battery Equivalent Circuit3/RConn1 -- Battery Equivalent Circuit2/LConn1

== system model1/Subsystem1/ControllerModel ==
  Average-Value DC-DC Converter : ee_lib/Semiconductors & Converters/Converters/Average-Value DC-DC Converter  control_option=ee.enum.converters.controlinput.dutycycle  converter_type=ee.enum.converters.dcdctype.buck  efficiency_option=ee.enum.converters.efficiency.constant  efficiency_fixed=100  i_vec=[0, 2, 5] A  efficiency_vec=[90, 95, 98]
      settings: InternalSimscapePortConfiguration="{\"Bottom\":[],\"Left\":[{\"id\":\"DutyCycle\",\"label\":\"DutyCycle\",\"type\":\"input\"},{\"id\":\"p1\",\"label\":\"1+\",\"type\":\"foundation.electrical.electrical\"},{\"id\":\"n1\",\"label\":\"1-\",\"type\":\"foundation.electrical.electrical\"}],\"Right\":[{\"id\":\"p2\",\"label\":\"2+\",\"type\":\"foundation.electrical.electrical\"},{\"id\":\"n2\",\"label\":\"2-\",\"type\":\"foundation.electrical.electrical\"}],\"Top\":[]}"
  Electrical Reference : fl_lib/Electrical/Electrical Elements/Electrical Reference
  DutyCycle : PMIOPort  Side=Left
  Con+ : PMIOPort  Port=2  Side=Left
  Con- : PMIOPort  Port=3  Side=Left
  Mot+ : PMIOPort  Port=4  Side=Right
  Mot- : PMIOPort  Port=5  Side=Right
  connections:
  Average-Value DC-DC Converter/RConn1 -- Mot+/RConn1
  Average-Value DC-DC Converter/LConn1 -- DutyCycle/RConn1
  Average-Value DC-DC Converter/LConn2 -- Con+/RConn1
  Average-Value DC-DC Converter/RConn2 -- Electrical Reference/LConn1 -- Mot-/RConn1
  Average-Value DC-DC Converter/LConn3 -- Con-/RConn1

== system model1/Subsystem1/Inclination Model ==
  Input : Inport
  1-D Lookup Table1 : Lookup_n-D  NumberOfTableDimensions=1  BreakpointsForDimension1=NewData{:,1}  Table=NewData{:,2}  InternalRulePriority=Speed  RndMeth=Simplest
  Bus Selector : BusSelector  OutputSignals=Distance (m),Velocity (km/h)
  Constant : Constant  Value=NewData{end,1}
  MATLAB Function1 : MATLAB Function  TreatAsAtomicUnit=on
  Scope3 : Scope  NumInputPorts=2
  Simulink-PS Converter3 : nesl_utility/Simulink-PS Converter  PhysicalDomain=network_engine_domain  SubClassName=ps_input  LeftPortType=input  RightPortType=output  PseudoPeriodic=off  Frequencies=[]  NoiseDistribution=none  NoiseParameters=[]  Unit=rad  AffineConversion=off  FilteringAndDerivatives=zero  SimscapeFilterOrder=1  InputFilterTimeConstant=0.001  UdotUserProvided=0
  Grad : PMIOPort  Side=Right
  wires:
  MATLAB Function1/1(position) -> 1-D Lookup Table1/1
  Constant/1 -> MATLAB Function1/2(s_track)
  Input/1 -> Bus Selector/1
  Bus Selector/2 -> Scope3/2  "<Velocity (km/h)>"
  Bus Selector/1 -> MATLAB Function1/1(s)  "<Distance (m)>"
  1-D Lookup Table1/1 -> Scope3/1, Simulink-PS Converter3/1
  connections:
  Simulink-PS Converter3/RConn1 -- Grad/RConn1

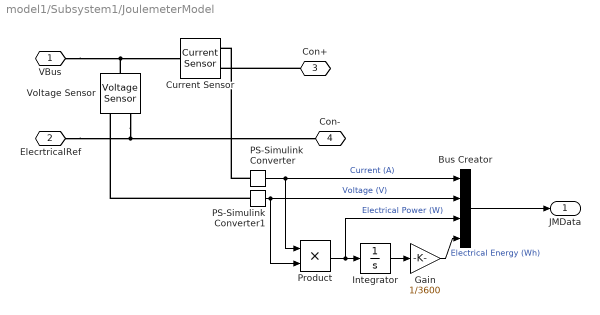
== system model1/Subsystem1/JoulemeterModel ==
  Bus Creator : BusCreator  Inputs=4
  Current Sensor : fl_lib/Electrical/Electrical Sensors/Current Sensor
  Gain : Gain  Gain=1/3600
  Integrator : Integrator
  PS-Simulink Converter : nesl_utility/PS-Simulink Converter  PhysicalDomain=network_engine_domain  SubClassName=ps_output  LeftPortType=input  RightPortType=output  PseudoPeriodic=off  Frequencies=[]  VectorFormat=1-D array  Unit=A  AffineConversion=off
  PS-Simulink Converter1 : nesl_utility/PS-Simulink Converter  PhysicalDomain=network_engine_domain  SubClassName=ps_output  LeftPortType=input  RightPortType=output  PseudoPeriodic=off  Frequencies=[]  VectorFormat=1-D array  Unit=V  AffineConversion=off
  Product : Product
  Voltage Sensor : fl_lib/Electrical/Electrical Sensors/Voltage Sensor
  VBus : PMIOPort  Side=Left
  ElecrtricalRef : PMIOPort  Port=2  Side=Left
  Con+ : PMIOPort  Port=3  Side=Right
  Con- : PMIOPort  Port=4  Side=Right
  JMData : Outport
  wires:
  PS-Simulink Converter/1 -> Product/1, Bus Creator/1  "Current (A)"
  PS-Simulink Converter1/1 -> Product/2, Bus Creator/2  "Voltage (V)"
  Bus Creator/1 -> JMData/1
  Product/1 -> Integrator/1, Bus Creator/3  "Electrical Power (W)"
  Gain/1 -> Bus Creator/4  "Electrical Energy (Wh)"
  Integrator/1 -> Gain/1
  connections:
  Voltage Sensor/LConn1 -- VBus/RConn1 -- Current Sensor/LConn1
  Voltage Sensor/RConn2 -- ElecrtricalRef/RConn1 -- Con-/RConn1
  PS-Simulink Converter1/LConn1 -- Voltage Sensor/RConn1
  PS-Simulink Converter/LConn1 -- Current Sensor/RConn1
  Con+/RConn1 -- Current Sensor/RConn2

== system model1/Subsystem1/PowertrainModel ==
  DC Motor : ee_lib/Electromechanical/Brushed Motors/DC Motor  Tag={'toolbox/physmod/elec/library/m/ee_lib_parts';'Electromechanical/Brushed_Motors/DC_Motor/Maxon/RE_65_388987_48.xml'}  field_option=ee.enum.field_option.pm  Rf=100 % Parameter not set Ohm  Lf=1 % Parameter not set H  Laf=0.15 % Parameter not set H  If0=0 % Parameter not set A  parameterization=ee.enum.dcparam_option.circuit_param  Ra=0.365 Ohm  La=0.161 mH  emf_or_torque=ee.enum.emf_or_torque.ki  Kv=12.88053 % Parameter estimated mV/rpm  Ki=123 mN*m/A  T_stall=0.24e-3 % Parameter not set N*m  w_max=19100 % Parameter not set rpm  w_rated=15000 % Parameter not set rpm  P_rated=0.08 % Parameter not set W  V_rated=1.5 % Parameter not set V  lam_param=ee.enum.lam_param.current  i_noload=0.289 A  V_i_noload=48 V  J=1340 g*cm^2  lam=0 % % Parameter not set mN*m/(rad/s)  speed0=0 % Parameter not set rpm  enable_fault_armature=simscape.enum.onoff.off  rev_faulted=1 / 3 % Parameter not set  G_faulted_armature=1e-5 % Parameter not set S  fault_trigger_armature=ee.enum.faults.faultTrigger.temporal  t_fault_armature=1 % Parameter not set s  max_permissible_current_armature=inf % Parameter not set A  t_fail_on_current_armature=1 % Parameter not set s  enable_fault_field=simscape.enum.onoff.off  G_faulted_field=1e-5 % Parameter not set S  fault_trigger_field=ee.enum.faults.faultTrigger.temporal  t_fault_field=1 % Parameter not set s  max_permissible_current_field=inf % Parameter not set A  t_fail_on_current_field=1 % Parameter not set s  fault_action=simscape.enum.assert.action.none  alpha=3.93e-3 % Parameter not set 1/K  Tmeas=25 % Parameter not set degC  thermal_mass=667.588357588358 % Parameter estimated J/K  initial_temperature=25 % Parameter not set degC
      settings: AttributesFormatString=Maxon:RE_65_388987_48
  Mechanical Rotational Reference : fl_lib/Mechanical/Rotational Elements/Mechanical Rotational Reference
  Simple Gear : sdl_lib/Gears/Simple Gear  ratio=RearGear/FrontGear  rotation_direction=sdl.enum.shaftOutputDirection.same  enable_faults=simscape.enum.onoff.off  efficiency_fault=0.05  fault_angles=pi / 12 rad  friction_model=sdl.enum.gear_efficiencies_load.off  T_noload=0.1 N*m  T_nom=5 N*m  efficiency_nom=0.8  efficiency=1  temperature_TLU=[280, 300, 320] K  load_TLU=[1, 5, 10] N*m  efficiency_TLU=[.95, .9, .85]  efficiency_TLU2=[.85, .8, .75; .95, .9, .85; .85, .8, .7]  w_thr=0.01 rad/s  pwr_thr=0.001 W  enable_backlash=false  hardstop_model=simscape.enum.hardstop.smooth  backlash_distance=1e-3 mm  r_base=0.1 m  transition=1e-4 mm  backlash_stiffness=1e6 N/m  backlash_damping=1e3 N*s/m  coeff_rest=0.7  v_tol=0.001 m/s  f_tol=0.001 N  mu_visc=[0, 0] N*m*s/rad  thermal_mass=50 J/K  temperature_specify=off  temperature_priority=High  temperature=300 K  temperature_nominal_specify=off  temperature_nominal_value=1  temperature_nominal_unit=K  x_backlash_specify=off  x_backlash_priority=None  x_backlash=0 mm  x_backlash_nominal_specify=off  x_backlash_nominal_value=1  x_backlash_nominal_unit=mm  f_hardstop_specify=off  f_hardstop_priority=None  f_hardstop=0 N  f_hardstop_nominal_specify=off  f_hardstop_nominal_value=1  f_hardstop_nominal_unit=N  v_backlash_specify=off  v_backlash_priority=None  v_backlash=0 m/s  v_backlash_nominal_specify=off  v_backlash_nominal_value=1  v_backlash_nominal_unit=m/s
  Unidirectional Clutch : sdl_lib/Clutches/Unidirectional Clutch  transmission_direction=sdl.enum.hubRingDirection.positive  initial_state_locked=sdl.enum.initial_lock.unlocked
      settings: InternalSimscapePortConfiguration="{\"Bottom\":[],\"Left\":[{\"id\":\"H\",\"label\":\"H\",\"type\":\"foundation.mechanical.rotational.rotational\"}],\"Right\":[{\"id\":\"R\",\"label\":\"R\",\"type\":\"foundation.mechanical.rotational.rotational\"}],\"Top\":[]}"
  Mot+ : PMIOPort  Side=Left
  Mot- : PMIOPort  Port=2  Side=Left
  Tire : PMIOPort  Port=3  Side=Right
  connections:
  Mechanical Rotational Reference/LConn1 -- DC Motor/RConn2
  DC Motor/RConn1 -- Mot-/RConn1
  DC Motor/LConn1 -- Mot+/RConn1
  DC Motor/LConn2 -- Simple Gear/LConn1
  Unidirectional Clutch/LConn1 -- Simple Gear/RConn1
  Unidirectional Clutch/RConn1 -- Tire/RConn1

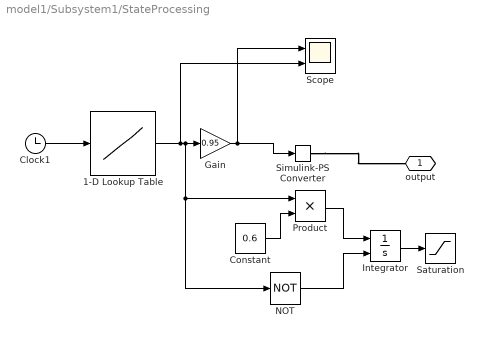
== system model1/Subsystem1/StateProcessing ==
  1-D Lookup Table : Lookup_n-D  NumberOfTableDimensions=1  BreakpointsForDimension1=finalatt{:,1}  IndexSearchMethod=Linear search  Table=finalatt{:,3}  InterpMethod=Flat  InternalRulePriority=Speed  RndMeth=Simplest
  Clock1 : Clock
  Constant : Constant  Value=0.6
  Gain : Gain  Gain=0.95
  Integrator : Integrator  ExternalReset=rising
  NOT : Logic  Operator=NOT  IconShape=distinctive  AllPortsSameDT=off  OutDataTypeStr=boolean
  Product : Product
  Saturation : Saturate  UpperLimit=0.95  LowerLimit=0
  Scope : Scope  NumInputPorts=2
  Simulink-PS Converter : nesl_utility/Simulink-PS Converter  PhysicalDomain=network_engine_domain  SubClassName=ps_input  LeftPortType=input  RightPortType=output  PseudoPeriodic=off  Frequencies=[]  NoiseDistribution=none  NoiseParameters=[]  Unit=1  AffineConversion=off  FilteringAndDerivatives=provide  SimscapeFilterOrder=1  InputFilterTimeConstant=0.001  UdotUserProvided=0
  output : PMIOPort  Side=Right
  wires:
  Clock1/1 -> 1-D Lookup Table/1
  1-D Lookup Table/1 -> Scope/2, Product/1, NOT/1, Gain/1
  Gain/1 -> Scope/1, Simulink-PS Converter/1
  Constant/1 -> Product/2
  Product/1 -> Integrator/1
  NOT/1 -> Integrator/2
  Integrator/1 -> Saturation/1
  connections:
  Simulink-PS Converter/RConn1 -- output/RConn1

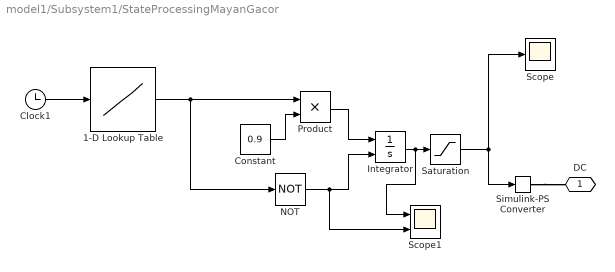
== system model1/Subsystem1/StateProcessingMayanGacor ==
  1-D Lookup Table : Lookup_n-D  NumberOfTableDimensions=1  BreakpointsForDimension1=finalatt{:,1}  IndexSearchMethod=Linear search  Table=finalatt{:,3}  InterpMethod=Flat  InternalRulePriority=Speed  RndMeth=Simplest
  Clock1 : Clock
  Constant : Constant  Value=0.9
  Integrator : Integrator  ExternalReset=rising
  NOT : Logic  Operator=NOT  IconShape=distinctive  AllPortsSameDT=off  OutDataTypeStr=boolean
  Product : Product
  Saturation : Saturate  UpperLimit=0.95  LowerLimit=0
  Scope : Scope
  Scope1 : Scope  NumInputPorts=2
  Simulink-PS Converter : nesl_utility/Simulink-PS Converter  PhysicalDomain=network_engine_domain  SubClassName=ps_input  LeftPortType=input  RightPortType=output  PseudoPeriodic=off  Frequencies=[]  NoiseDistribution=none  NoiseParameters=[]  Unit=1  AffineConversion=off  FilteringAndDerivatives=provide  SimscapeFilterOrder=1  InputFilterTimeConstant=0.001  UdotUserProvided=0
  DC : PMIOPort  Side=Right
  wires:
  Integrator/1 -> Scope1/1, Saturation/1
  NOT/1 -> Scope1/2, Integrator/2
  1-D Lookup Table/1 -> Product/1, NOT/1
  Constant/1 -> Product/2
  Product/1 -> Integrator/1
  Clock1/1 -> 1-D Lookup Table/1
  Saturation/1 -> Simulink-PS Converter/1, Scope/1
  connections:
  Simulink-PS Converter/RConn1 -- DC/RConn1

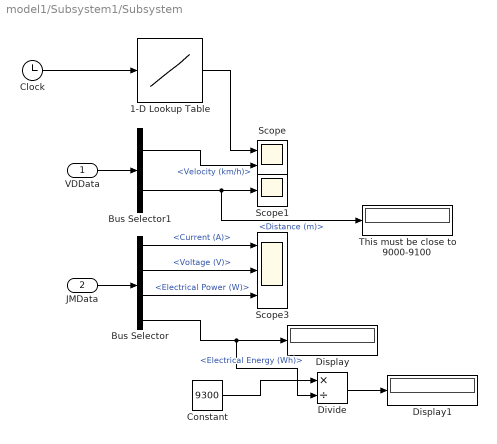
== system model1/Subsystem1/Subsystem ==
  VDData : Inport
  JMData : Inport  Port=2
  1-D Lookup Table : Lookup_n-D  NumberOfTableDimensions=1  BreakpointsForDimension1=finalatt{:,1}  Table=finalatt{:,2}  InternalRulePriority=Speed  RndMeth=Simplest
  Bus Selector : BusSelector  OutputSignals=Current (A),Voltage (V),Electrical Power (W),Electrical Energy (Wh)
  Bus Selector1 : BusSelector  OutputSignals=Velocity (km/h),Distance (m)
  Clock : Clock
  Constant : Constant  Value=9300
  Display : Display
  Display1 : Display
  Divide : Product  Inputs=*/
  Scope : Scope  NumInputPorts=2
  Scope1 : Scope
  Scope3 : Scope  NumInputPorts=3
  This must be close to 9000-9100 : Display
  wires:
  JMData/1 -> Bus Selector/1
  VDData/1 -> Bus Selector1/1
  Bus Selector1/1 -> Scope/2  "<Velocity (km/h)>"
  Bus Selector1/2 -> This must be close to 9000-9100/1, Scope1/1  "<Distance (m)>"
  Bus Selector/3 -> Scope3/3  "<Electrical Power (W)>"
  Bus Selector/2 -> Scope3/2  "<Voltage (V)>"
  Bus Selector/1 -> Scope3/1  "<Current (A)>"
  Bus Selector/4 -> Divide/2, Display/1  "<Electrical Energy (Wh)>"
  Clock/1 -> 1-D Lookup Table/1
  1-D Lookup Table/1 -> Scope/1
  Constant/1 -> Divide/1
  Divide/1 -> Display1/1

== system model1/Subsystem1/Subsystem1 ==
  Velocity : Inport
  1-D Lookup Table2 : Lookup_n-D  NumberOfTableDimensions=1  BreakpointsForDimension1=finalatt{:,1}  Table=finalatt{:,3}  InterpMethod=Flat  InternalRulePriority=Speed  RndMeth=Simplest
  Bus Selector : BusSelector  OutputSignals=Velocity (km/h)
  Clock1 : Clock
  Subsystem : Subsystem
  DutyCycle : PMIOPort  Side=Right
  wires:
  1-D Lookup Table2/1 -> Subsystem/1(control)
  Clock1/1 -> 1-D Lookup Table2/1
  Velocity/1 -> Bus Selector/1
  Bus Selector/1 -> Subsystem/2(velocity)  "<Velocity (km/h)>"
  connections:
  DutyCycle/RConn1 -- Subsystem/RConn1
